simulink model "FCEvReferenceApplication"  (R2022a)
settings: Solver=VariableStepAuto  StartTime=0  StopTime=2474  RelTol=1e-3  EnableMultiTasking=on
undefined symbols (not defined in the file or in its folder): GenerateMappedFuelCellCalibrations
libraries: autolibshared x2
settings Model: DataDictionary=VehicleConfig.sldd  ModifiedByFormat=The MathWorks, Inc.  SimulationMode=accelerator  PauseTimes=0  Creator=The MathWorks, Inc.  LastModifiedBy=The MathWorks, Inc.
settings SolverCC: MaxConsecutiveMinStep=3  ZeroCrossAlgorithm=Adaptive  AlgebraicLoopSolver=TrustRegion  AutoInsertRateTranBlk=on  DecoupledContinuousIntegration=on  MinimalZcImpactIntegration=on  MaxZcPerStep=1
settings DataIOCC: SaveOutput=off  DSMLogging=off  SaveTime=off  ReturnWorkspaceOutputs=off
settings DebuggingCC: UnderspecifiedInitializationDetection=Classic  MergeDetectMultiDrivingBlocksExec=none  IgnoredZcDiagnostic=none  UnconnectedInputMsg=warning  UnconnectedOutputMsg=warning  UnconnectedLineMsg=warning  ModelReferenceExtraNoncontSigs=none  PregeneratedLibrarySubsystemCodeDiagnostic=none  SFMachineParentedDataDiag=warning  ArithmeticOperatorsInVariantConditions=warning
settings ModelReferenceCC: UpdateModelReferenceTargets=IfOutOfDate  ModelReferenceMinAlgLoopOccurrences=on  PropagateSignalLabelsOutOfModel=off
settings SFSimCC: SimUseLocalCustomCode=off
settings RTWCC: RTWUseLocalCustomCode=off  DLArmComputeVersion=19.05
settings CodeAppCC: StateflowObjectComments=on
settings GRTTargetCC: TargetLangStandard=C89/C90 (ANSI)
settings ConfigComp: CovMetricSettings=dsw  CovSaveCumulativeToWorkspaceVar=on  CovSaveSingleToWorkspaceVar=on  CovExternalEMLEnable=off

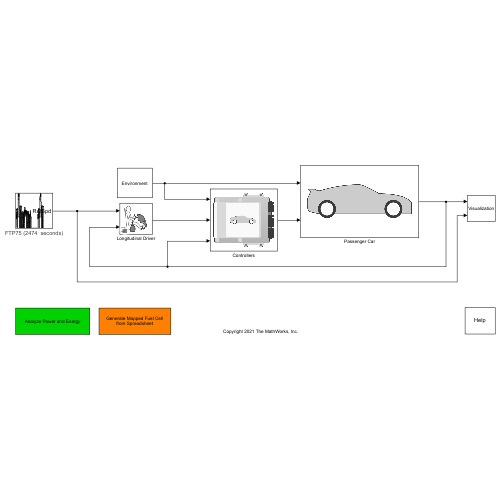
[thumbnail: Simulink's stored preview of the top-level diagram]
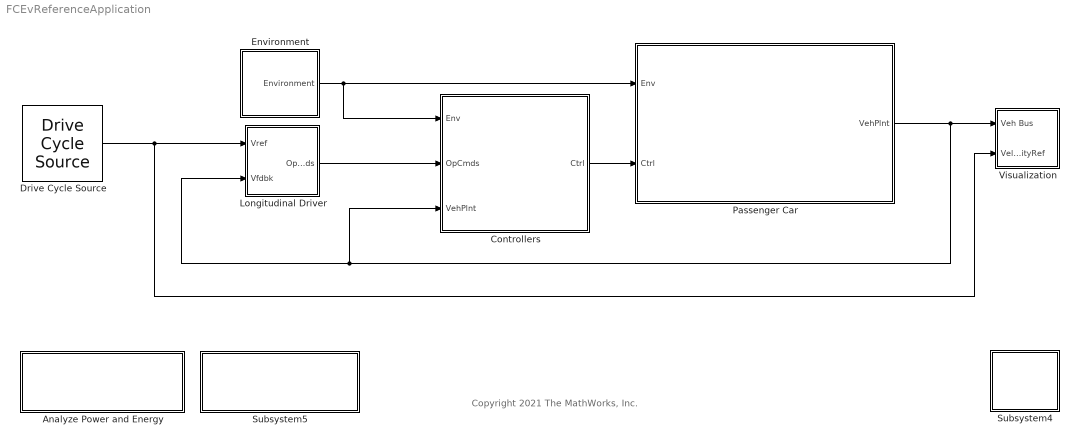
== system FCEvReferenceApplication ==
  note: Copyright 2021 The MathWorks, Inc.
  Analyze Power and Energy : Subsystem
      settings: OpenFcn=edit GenerateEnergyReport
      mask Display: disp(getString(message('autoblks:autoblkVehMask:powAndEne')))
  Controllers : Subsystem
      mask Display: image('SystemControllers.png','center')
  Drive Cycle Source : autolibshared/Drive Cycle Source  cycleVar=FTP75  fileVar=L:\Bauto\matlab\test\toolbox\shared\autoblks\scenario\adac.txt  tfinal="2474  seconds"  cycleRepeat=off  outAccPort=off  outGearPort=off  gearList=No gear data  t_wot1=1  xdot_woto=0  xdot_wot1=26.8  t_wot2=30  xdot_wot2=0  t_wotend=40  srcUnit=m/s  outUnit=m/s  srcAccUnit=m/s/s  outAccUnit=m/s^2  dt=0  aMode=1  faultOption=off  velBnd=2  velBndUnit=mph  inUnit=m/s  timeBnd=1  failOption=off  stopSim=off  maxFaultCnt=10  maxFaultTime=2  maxTotFaultTime=15  traceOption=off  dtTrace=1  traceWindow=10  lastDCname=FTP75  lastOutUnit=mph  lastDT=0  lastTB=1  lastSB=2  forceCalcBound=off
      settings: SourceProductBaseCode=PW,DR,MT,VE
  Environment : Subsystem
      mask Display: disp(getString(message('autoblks:autoblkVehMask:environ')))
  Longitudinal Driver : Subsystem  Variant=on  VariantControlMode=label  VariantControl=Variant1  LabelModeActiveChoice=0
      mask Display:
      | if strcmp('1',get_param(gcb,'ActiveVariant'))
      |     disp('Open Loop')
      | else
      |     image('LongitudinalDriver.png','center');
      | end
  Passenger Car : Subsystem
      mask Display: image('PassengerVehicle.png','center')
  Subsystem4 : Subsystem
      settings: OpenFcn=helpview([docroot,'/toolbox/autoblks/helptargets.map'], 'fcev_refapp')
      mask Display: disp(getString(message('autoblks:autoblkVehMask:help')))
  Subsystem5 : Subsystem  LoadFcn=GenerateMappedFuelCellCalibrations(gcb, 'CheckMBCLicense');  mask(Generate Mapped Fuel Cell from Spreadsheet){SpreadsheetFileName=FuelCellPerformanceData.xlsx, MBCProjectName=MappedFuelCell.mat, CageFileName=MappedFuelCell.cag, MappedFCellMdlRefName=FCElectricPlant}
      mask prompts: SpreadsheetFileName "autoblks:autoblkMappedFuelCellMask:mapSheetFile"; MBCProjectName "autoblks:autoblkMappedFuelCellMask:mbcProj"; CageFileName "autoblks:autoblkMappedFuelCellMask:cageFile"; MappedFCellMdlRefName "autoblks:autoblkMappedFuelCellMask:mappedEng"
      mask help: autoblks:autoblkMappedFuelCellMask:descSheet
      mask init:
      | GenerateMappedFuelCellCalibrations(gcb, 'Init');
      settings: OpenFcn=open_system(gcb, 'mask')
      mask Help: helpview([docroot,'/toolbox/autoblks/helptargets.map'], 'fcev_mapped_spreadsheet')
      mask DialogControl DescTextVar Prompt: autoblks:autoblkMappedFuelCellMask:descSheet
      mask DialogControl MBCHyperlink Prompt: autoblks:autoblkMappedFuelCellMask:reqOpt
      mask DialogControl MBCHyperlink Callback: helpview([docroot,'/toolbox/autoblks/helptargets.map'], 'siengine_dyno_refapp')
      mask DialogControl Container3 Prompt: autoblks:autoblkMappedFuelCellMask:step1
      mask DialogControl SpreadsheetFileName Prompt: Spreadsheet file:
      mask DialogControl SpreadsheetFileNameSelect Prompt: autoblks:autoblkMappedFuelCellMask:ellipsis
      mask DialogControl SpreadsheetFileNameSelect Callback: GenerateMappedFuelCellCalibrations(gcb, 'SpreadsheetFileNameSelect');
      mask DialogControl GenMappedFCellCalButton Prompt: autoblks:autoblkMappedFuelCellMask:fcellCal
      mask DialogControl GenMappedFCellCalButton Callback: GenerateMappedFuelCellCalibrations(gcb, 'GenMappedFCellCalButton');
      mask DialogControl MBCProjectName Prompt: MBC project name:
      mask DialogControl CageFileName Prompt: CAGE file name:
      mask DialogControl Container4 Prompt: autoblks:autoblkMappedFuelCellMask:step2
      mask DialogControl ApplyCalMappedFCellButton Prompt: autoblks:autoblkMappedFuelCellMask:applyCal
      mask DialogControl ApplyCalMappedFCellButton Callback: GenerateMappedFuelCellCalibrations(gcb, 'ApplyCalMappedFCellButton');
      mask Display: disp(getString(message('autoblks:autoblkMappedFuelCellMask:mapSpreadLabel')))
  Visualization : Subsystem
      mask Display: disp(getString(message('autoblks:autoblkVehMask:visual')))
  wires:
  Longitudinal Driver/1(" OpCmds") -> Controllers/2(OpCmds)
  Drive Cycle Source/1 -> Longitudinal Driver/1("Vref "), Visualization/2(VelocityRef)
  Environment/1(Environment) -> Controllers/1(Env), Passenger Car/1(Env)
  Controllers/1(Ctrl) -> Passenger Car/2(Ctrl)
  Passenger Car/1(VehPlnt) -> Controllers/3(VehPlnt), Longitudinal Driver/2("Vfdbk "), Visualization/1(Veh Bus)

== system FCEvReferenceApplication/Analyze Power and Energy ==

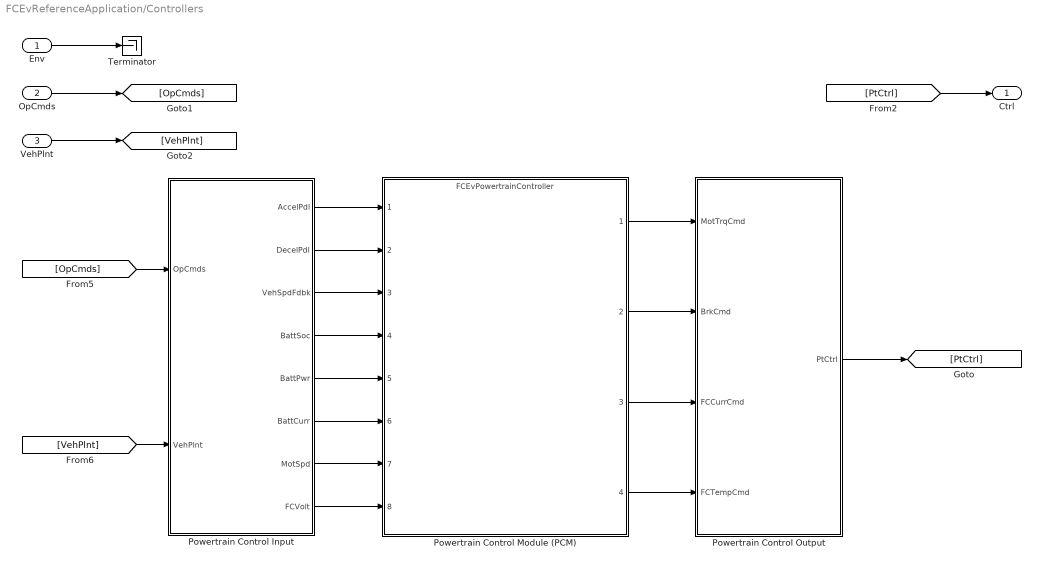
== system FCEvReferenceApplication/Controllers ==
  Env : Inport
  OpCmds : Inport  Port=2
  VehPlnt : Inport  Port=3
  Powertrain Control Input : Subsystem
  Powertrain Control Module (PCM) : ModelReference  ModelNameDialog=FCEvPowertrainController.slx  ModelReferenceVersion=4.1
  Powertrain Control Output : Subsystem
  Terminator : Terminator
  Ctrl : Outport  VectorParamsAs1DForOutWhenUnconnected=off
  wires:
  [OpCmds] -> Powertrain Control Input/1(OpCmds)
  Powertrain Control Input/6(BattCurr) -> Powertrain Control Module (PCM)/6
  Powertrain Control Module (PCM)/4 -> Powertrain Control Output/4(FCTempCmd)
  VehPlnt/1 -> [VehPlnt]
  Powertrain Control Input/2(DecelPdl) -> Powertrain Control Module (PCM)/2
  Powertrain Control Input/3(VehSpdFdbk) -> Powertrain Control Module (PCM)/3
  Powertrain Control Input/5(BattPwr) -> Powertrain Control Module (PCM)/5
  Powertrain Control Input/8(FCVolt) -> Powertrain Control Module (PCM)/8
  [PtCtrl] -> Ctrl/1
  [VehPlnt] -> Powertrain Control Input/2(VehPlnt)
  OpCmds/1 -> [OpCmds]
  Powertrain Control Input/4(BattSoc) -> Powertrain Control Module (PCM)/4
  Powertrain Control Module (PCM)/3 -> Powertrain Control Output/3(FCCurrCmd)
  Powertrain Control Module (PCM)/1 -> Powertrain Control Output/1(MotTrqCmd)
  Powertrain Control Module (PCM)/2 -> Powertrain Control Output/2(BrkCmd)
  Powertrain Control Input/7(MotSpd) -> Powertrain Control Module (PCM)/7
  Env/1 -> Terminator/1
  Powertrain Control Input/1(AccelPdl) -> Powertrain Control Module (PCM)/1
  Powertrain Control Output/1(PtCtrl) -> [PtCtrl]

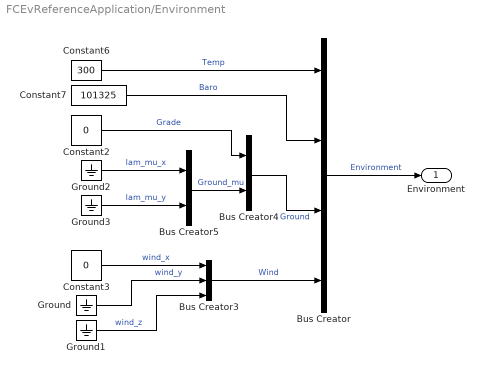
== system FCEvReferenceApplication/Environment ==
  Bus Creator : BusCreator  Inputs=4
  Bus Creator3 : BusCreator  Inputs=3
  Bus Creator4 : BusCreator  Inputs=2
  Bus Creator5 : BusCreator  Inputs=2
  Constant2 : Constant  Value=0
  Constant3 : Constant  Value=0
  Constant6 : Constant  Value=300
  Constant7 : Constant  Value=101325
  Ground{,1..3} (4 alike) : Ground
  Environment : Outport  VectorParamsAs1DForOutWhenUnconnected=off
  wires:
  Ground2/1 -> Bus Creator5/1  "lam_mu_x"
  Ground3/1 -> Bus Creator5/2  "lam_mu_y"
  Bus Creator5/1 -> Bus Creator4/2  "Ground_mu"
  Bus Creator4/1 -> Bus Creator/3  "Ground"
  Bus Creator3/1 -> Bus Creator/4  "Wind"
  Constant3/1 -> Bus Creator3/1  "wind_x"
  Ground/1 -> Bus Creator3/2  "wind_y"
  Ground1/1 -> Bus Creator3/3  "wind_z"
  Constant6/1 -> Bus Creator/1  "Temp"
  Constant2/1 -> Bus Creator4/1  "Grade"
  Bus Creator/1 -> Environment/1  "Environment"
  Constant7/1 -> Bus Creator/2  "Baro"

== system FCEvReferenceApplication/Longitudinal Driver ==
  note: To switch variants, right-click on this subsystem (from one level above) and chose:
      | Variant, Active choice, <your selection>
  "Vref " : Inport
  "Vfdbk " : Inport  Port=2
  Longitudinal Driver : Subsystem  VariantControl=0
      mask Display: image('LongitudinalDriver.png', 'center')
  Open Loop : Subsystem  VariantControl=1
      mask Display: disp('Open Loop')
  " OpCmds" : Outport  VectorParamsAs1DForOutWhenUnconnected=off

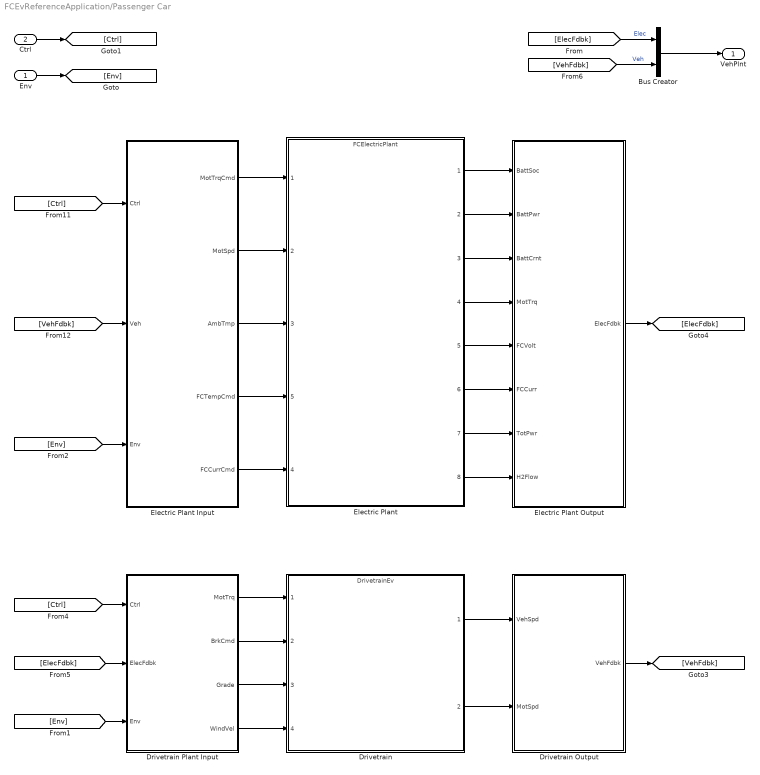
== system FCEvReferenceApplication/Passenger Car ==
  Env : Inport
  Ctrl : Inport  Port=2
  Bus Creator : BusCreator  Inputs=2
  Drivetrain : ModelReference  ModelNameDialog=DrivetrainEv.slx  ModelReferenceVersion=6.1
  Drivetrain Output : Subsystem
  Drivetrain Plant Input : Subsystem
  Electric Plant : ModelReference  ModelNameDialog=FCElectricPlant.slx  ModelReferenceVersion=4.151
      settings: PortSchema="{\"entries\":[{\"content\":{\"sides\":[{\"content\":{\"connectorIds\":[\"In1\",\"In2\",\"In3\",\"In5\",\"In4\"]},\"type\":\"ConnectorPlacement.EquallySpacedRectSide\",\"uuid\":\"252331aa-c2e1-4212-91c7-54a4f8807c1b\"},{\"content\":{\"connectorIds\":[\"Out1\",\"Out2\",\"Out3\",\"Out4\",\"Out5\",\"Out6\",\"Out7\",\"Out8\"],\"side\":\"RIGHT\"},\"type\":\"ConnectorPlacement.EquallySpacedRectSide\",\"uuid\":\"96a2e807-7b6e-43c6-b371-83afbf277557\"},{\"content\":{\"connectorIds\":[],\"side\":\"TOP\"},\"type\":\"ConnectorPlacement.EquallySpacedRectSide\",\"uuid\":\"573edb4a-38fa-4d49-8fd7-93dca65813a5\"}]},\"type\":\"ConnectorPlacement.EquallySpacedConnector\",\"uuid\":\"acfa41e8-7930-436b-acd7-e14a4a7fb9aa\"}],\"packageUris\":[\"http://schema.mathworks.com/mf0/Connector/R2020b\"],\"version\":\"1.0\"}"
  Electric Plant Input : Subsystem
  Electric Plant Output : Subsystem
  VehPlnt : Outport  VectorParamsAs1DForOutWhenUnconnected=off
  wires:
  Electric Plant/1 -> Electric Plant Output/1(BattSoc)
  Env/1 -> [Env]
  Electric Plant/6 -> Electric Plant Output/6(FCCurr)
  Electric Plant/5 -> Electric Plant Output/5(FCVolt)
  Electric Plant/3 -> Electric Plant Output/3(BattCrnt)
  Electric Plant/4 -> Electric Plant Output/4(MotTrq)
  Bus Creator/1 -> VehPlnt/1
  [ElecFdbk] -> Bus Creator/1  "Elec"
  Electric Plant Output/1(ElecFdbk) -> [ElecFdbk]
  [Env] -> Electric Plant Input/3(Env)
  Electric Plant Input/4(FCTempCmd) -> Electric Plant/5
  Electric Plant Input/2(MotSpd) -> Electric Plant/2
  Electric Plant Input/1(MotTrqCmd) -> Electric Plant/1
  Electric Plant/2 -> Electric Plant Output/2(BattPwr)
  [VehFdbk] -> Bus Creator/2  "Veh"
  Electric Plant Input/5(FCCurrCmd) -> Electric Plant/4
  [Ctrl] -> Electric Plant Input/1(Ctrl)
  Ctrl/1 -> [Ctrl]
  [VehFdbk] -> Electric Plant Input/2(Veh)
  Electric Plant Input/3(AmbTmp) -> Electric Plant/3
  Drivetrain/1 -> Drivetrain Output/1(VehSpd)
  Drivetrain Plant Input/2(BrkCmd) -> Drivetrain/2
  Drivetrain Output/1(VehFdbk) -> [VehFdbk]
  [Ctrl] -> Drivetrain Plant Input/1(Ctrl)
  Drivetrain Plant Input/1(MotTrq) -> Drivetrain/1
  [Env] -> Drivetrain Plant Input/3(Env)
  Drivetrain Plant Input/4(WindVel) -> Drivetrain/4
  Drivetrain Plant Input/3(Grade) -> Drivetrain/3
  Drivetrain/2 -> Drivetrain Output/2(MotSpd)
  [ElecFdbk] -> Drivetrain Plant Input/2(ElecFdbk)
  Electric Plant/7 -> Electric Plant Output/7(TotPwr)
  Electric Plant/8 -> Electric Plant Output/8(H2Flow)

== system FCEvReferenceApplication/Subsystem4 ==

== system FCEvReferenceApplication/Subsystem5 ==

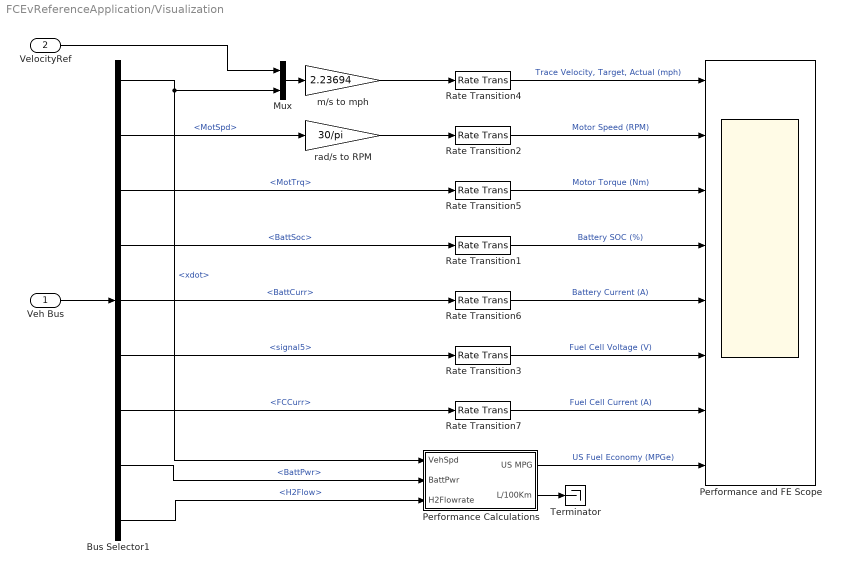
== system FCEvReferenceApplication/Visualization ==
  Veh Bus : Inport
  VelocityRef : Inport  Port=2
  Bus Selector1 : BusSelector  OutputSignals=Veh.xdot,Veh.MotSpd,Elec.MotTrq,Elec.BattSoc,Elec.BattCurr,Elec.signal5,Elec.FCCurr,Elec.BattPwr,Elec.H2Flow
  Mux : Mux  Inputs=2
  Performance Calculations : Subsystem
  Performance and FE Scope : Scope  NumInputPorts=8
  Rate Transition{1..7} (7 alike) : RateTransition  Deterministic=off
  Terminator : Terminator
  m/s to mph : Gain  Gain=2.23694
  rad/s to RPM : Gain  Gain=30/pi
  wires:
  Veh Bus/1 -> Bus Selector1/1
  Bus Selector1/1 -> Performance Calculations/1(VehSpd), Mux/2  "<xdot>"
  Mux/1 -> m/s to mph/1
  Performance Calculations/1(US MPG) -> Performance and FE Scope/8  "US Fuel Economy (MPGe)"
  Performance Calculations/2(L/100Km) -> Terminator/1
  m/s to mph/1 -> Rate Transition4/1
  Bus Selector1/4 -> Rate Transition1/1  "<BattSoc>"
  VelocityRef/1 -> Mux/1
  Rate Transition1/1 -> Performance and FE Scope/4  "Battery SOC (%)"
  Rate Transition2/1 -> Performance and FE Scope/2  "Motor Speed (RPM)"
  Rate Transition4/1 -> Performance and FE Scope/1  "Trace Velocity, Target, Actual (mph)"
  Bus Selector1/2 -> rad/s to RPM/1  "<MotSpd>"
  Bus Selector1/8 -> Performance Calculations/2(BattPwr)  "<BattPwr>"
  rad/s to RPM/1 -> Rate Transition2/1
  Bus Selector1/3 -> Rate Transition5/1  "<MotTrq>"
  Rate Transition5/1 -> Performance and FE Scope/3  "Motor Torque (Nm)"
  Rate Transition6/1 -> Performance and FE Scope/5  "Battery Current (A)"
  Bus Selector1/5 -> Rate Transition6/1  "<BattCurr>"
  Bus Selector1/9 -> Performance Calculations/3(H2Flowrate)  "<H2Flow>"
  Bus Selector1/7 -> Rate Transition7/1  "<FCCurr>"
  Rate Transition7/1 -> Performance and FE Scope/7  "Fuel Cell Current (A)"
  Bus Selector1/6 -> Rate Transition3/1  "<signal5>"
  Rate Transition3/1 -> Performance and FE Scope/6  "Fuel Cell Voltage (V)"

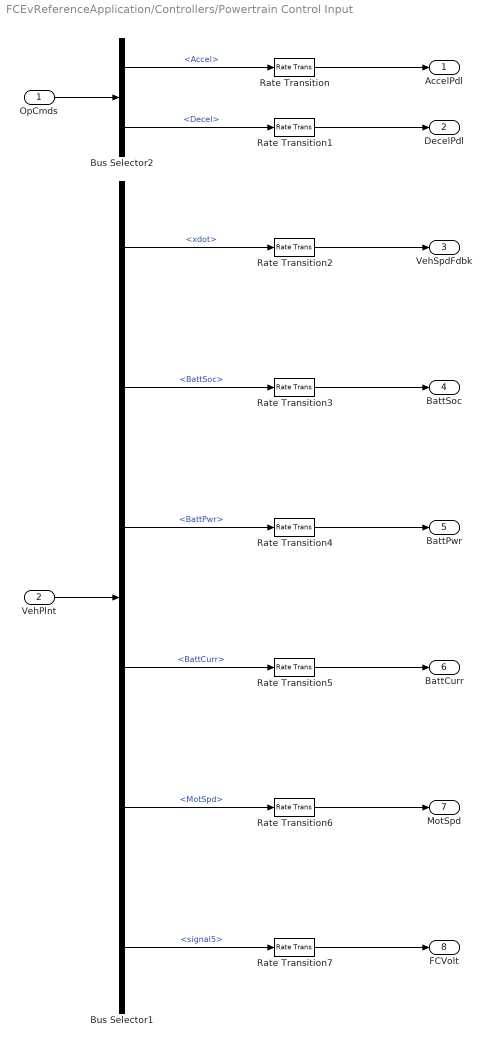
== system FCEvReferenceApplication/Controllers/Powertrain Control Input ==
  OpCmds : Inport
  VehPlnt : Inport  Port=2
  Bus Selector1 : BusSelector  OutputSignals=Veh.xdot,Elec.BattSoc,Elec.BattPwr,Elec.BattCurr,Veh.MotSpd,Elec.signal5
  Bus Selector2 : BusSelector  OutputSignals=Accel,Decel
  Rate Transition{,1..7} (8 alike) : RateTransition  Deterministic=off
  AccelPdl : Outport  VectorParamsAs1DForOutWhenUnconnected=off
  DecelPdl : Outport  Port=2  VectorParamsAs1DForOutWhenUnconnected=off
  VehSpdFdbk : Outport  Port=3  VectorParamsAs1DForOutWhenUnconnected=off
  BattSoc : Outport  Port=4  VectorParamsAs1DForOutWhenUnconnected=off
  BattPwr : Outport  Port=5  VectorParamsAs1DForOutWhenUnconnected=off
  BattCurr : Outport  Port=6  VectorParamsAs1DForOutWhenUnconnected=off
  MotSpd : Outport  Port=7  VectorParamsAs1DForOutWhenUnconnected=off
  FCVolt : Outport  Port=8  VectorParamsAs1DForOutWhenUnconnected=off
  wires:
  OpCmds/1 -> Bus Selector2/1
  VehPlnt/1 -> Bus Selector1/1
  Bus Selector2/1 -> Rate Transition/1  "<Accel>"
  Bus Selector2/2 -> Rate Transition1/1  "<Decel>"
  Bus Selector1/1 -> Rate Transition2/1  "<xdot>"
  Bus Selector1/2 -> Rate Transition3/1  "<BattSoc>"
  Bus Selector1/3 -> Rate Transition4/1  "<BattPwr>"
  Bus Selector1/4 -> Rate Transition5/1  "<BattCurr>"
  Bus Selector1/5 -> Rate Transition6/1  "<MotSpd>"
  Rate Transition/1 -> AccelPdl/1
  Rate Transition1/1 -> DecelPdl/1
  Rate Transition2/1 -> VehSpdFdbk/1
  Rate Transition3/1 -> BattSoc/1
  Rate Transition4/1 -> BattPwr/1
  Rate Transition5/1 -> BattCurr/1
  Rate Transition6/1 -> MotSpd/1
  Rate Transition7/1 -> FCVolt/1
  Bus Selector1/6 -> Rate Transition7/1  "<signal5>"

== system FCEvReferenceApplication/Controllers/Powertrain Control Output ==
  MotTrqCmd : Inport
  BrkCmd : Inport  Port=2
  FCCurrCmd : Inport  Port=3
  FCTempCmd : Inport  Port=4
  Bus Creator : BusCreator  Inputs=4
  PtCtrl : Outport  VectorParamsAs1DForOutWhenUnconnected=off
  wires:
  BrkCmd/1 -> Bus Creator/2  "BrkCmd"
  Bus Creator/1 -> PtCtrl/1  "PtCtrl"
  MotTrqCmd/1 -> Bus Creator/1  "MotTrqCmd"
  FCCurrCmd/1 -> Bus Creator/3  "FCCurrCmd"
  FCTempCmd/1 -> Bus Creator/4  "FCTempCmd"

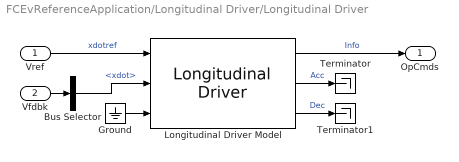
== system FCEvReferenceApplication/Longitudinal Driver/Longitudinal Driver ==
  Vref : Inport
  Vfdbk : Inport  Port=2
  Bus Selector : BusSelector  OutputSignals=Veh.xdot
  Ground : Ground
  Longitudinal Driver Model : autolibshared/Longitudinal Driver  extAccelOvr=off  extDecelOvr=off  extAccelHld=off  extDecelHld=off  extAccelZero=off  extDecelZero=off  cntrlType=Predictive  shftType=Reverse, Neutral, Drive  velUnits=m/s  gearOut=off  Kp=1  Ki=1  Kff=0  Kg=0  VehVelVec=[0 100]  KffVec=[.1 .1]  KpVec=[10 10]  KiVec=[5 5]  KgVec=[0 0]  m=1500  Kpt=10000  tau=0.12  L=4  aR=160  bR=1  cR=0.36  g=9.81  vnom=1  Kaw=0  tauerr=0  tauPt=2  GearInit=0  tShift=.1  pdlVec=[0.1 0.4 0.5 0.9]  upShftTbl=[-1 12.9375 26.4375 39.9375 51.18749999999999 62.4375 72.84375 83.25;-1 16.3125 29.8125 43.3125 54.5624 65.8125 76.78125 87.75;-1 19.6875 33.1875 46.68749999999999 57.9375 69.1875 80.71875 92.25;-1 33 52.5 77.25 100.5 138.75 161.875 185]  dwnShftTbl=[1 9.5625 23.0625 36.5625 47.8125 59.0625 68.90625 78.75;1 12.9375 26.4375 39.9375 51.18749999999999 62.4375 72.84375 83.25;1 16.3125 29.8125 43.3125 54.562499 65.8125 76.78125 87.75;1 19.6875 33.1875 46.68749999999999 57.9375 69.1875 80.71875 92.25]  tClutch=.5  tRev=.5  tPark=120  aMode=1  UpGearVec="[0  1  2  3  4  5  6  7]"  DownGearVec="[1  2  3  4  5  6  7  8]"
      settings: SourceProductBaseCode=PW,DR,MT,VE
  Terminator : Terminator
  Terminator1 : Terminator
  OpCmds : Outport  VectorParamsAs1DForOutWhenUnconnected=off
  wires:
  Bus Selector/1 -> Longitudinal Driver Model/2  "<xdot>"
  Vref/1 -> Longitudinal Driver Model/1  "xdotref"
  Vfdbk/1 -> Bus Selector/1
  Longitudinal Driver Model/2 -> Terminator/1  "Acc"
  Longitudinal Driver Model/3 -> Terminator1/1  "Dec"
  Ground/1 -> Longitudinal Driver Model/3
  Longitudinal Driver Model/1 -> OpCmds/1  "Info"

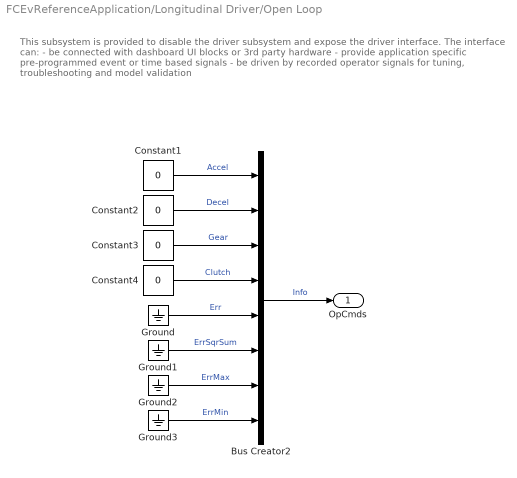
== system FCEvReferenceApplication/Longitudinal Driver/Open Loop ==
  note: This subsystem is provided to disable the driver subsystem and expose the driver interface.
      |
      | The interface can:
      | - be connected with dashboard UI blocks or 3rd party hardware
      | - provide application specific pre-programmed event or time based signals
      | - be driven by recorded operator signals for tuning, troubleshooting and model validation
  Bus Creator2 : BusCreator  Inputs=8
  Constant{1..4} (4 alike) : Constant  Value=0
  Ground{,1..3} (4 alike) : Ground
  OpCmds : Outport  VectorParamsAs1DForOutWhenUnconnected=off
  wires:
  Ground3/1 -> Bus Creator2/8  "ErrMin"
  Ground1/1 -> Bus Creator2/6  "ErrSqrSum"
  Bus Creator2/1 -> OpCmds/1  "Info"
  Ground2/1 -> Bus Creator2/7  "ErrMax"
  Constant1/1 -> Bus Creator2/1  "Accel"
  Constant3/1 -> Bus Creator2/3  "Gear"
  Constant2/1 -> Bus Creator2/2  "Decel"
  Ground/1 -> Bus Creator2/5  "Err"
  Constant4/1 -> Bus Creator2/4  "Clutch"

== system FCEvReferenceApplication/Passenger Car/Drivetrain Output ==
  VehSpd : Inport
  MotSpd : Inport  Port=2
  Bus Creator1 : BusCreator  Inputs=2
  VehFdbk : Outport  VectorParamsAs1DForOutWhenUnconnected=off
  wires:
  Bus Creator1/1 -> VehFdbk/1  "VehFdbk"
  VehSpd/1 -> Bus Creator1/1
  MotSpd/1 -> Bus Creator1/2  "MotSpd"

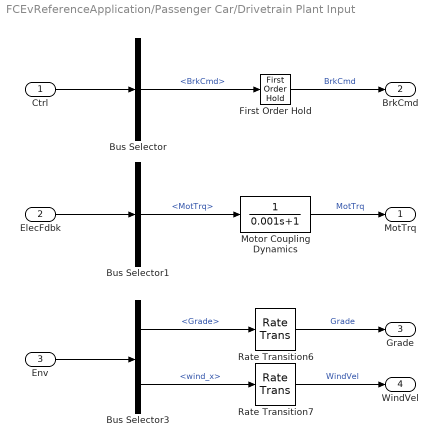
== system FCEvReferenceApplication/Passenger Car/Drivetrain Plant Input ==
  Ctrl : Inport
  ElecFdbk : Inport  Port=2
  Env : Inport  Port=3
  Bus Selector : BusSelector  OutputSignals=BrkCmd
  Bus Selector1 : BusSelector  OutputSignals=MotTrq
  Bus Selector3 : BusSelector  OutputSignals=Ground.Grade,Wind.wind_x
  First Order Hold : FirstOrderHold  ErrorTolerance=inf
  Motor Coupling Dynamics : TransferFcn  Denominator=[0.001 1]
  Rate Transition6 : RateTransition  Deterministic=off
  Rate Transition7 : RateTransition  Deterministic=off
  MotTrq : Outport  VectorParamsAs1DForOutWhenUnconnected=off
  BrkCmd : Outport  Port=2  VectorParamsAs1DForOutWhenUnconnected=off
  Grade : Outport  Port=3  VectorParamsAs1DForOutWhenUnconnected=off
  WindVel : Outport  Port=4  VectorParamsAs1DForOutWhenUnconnected=off
  wires:
  Ctrl/1 -> Bus Selector/1
  Bus Selector/1 -> First Order Hold/1  "<BrkCmd>"
  First Order Hold/1 -> BrkCmd/1  "BrkCmd"
  ElecFdbk/1 -> Bus Selector1/1
  Bus Selector1/1 -> Motor Coupling Dynamics/1  "<MotTrq>"
  Env/1 -> Bus Selector3/1
  Rate Transition6/1 -> Grade/1  "Grade"
  Rate Transition7/1 -> WindVel/1  "WindVel"
  Bus Selector3/1 -> Rate Transition6/1  "<Grade>"
  Bus Selector3/2 -> Rate Transition7/1  "<wind_x>"
  Motor Coupling Dynamics/1 -> MotTrq/1  "MotTrq"

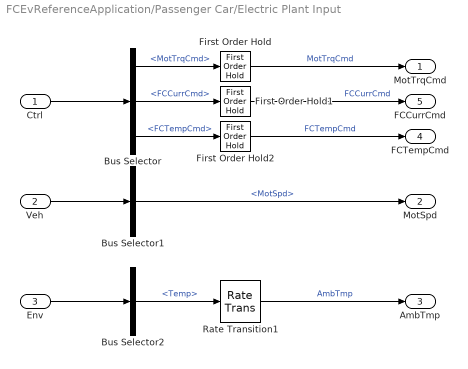
== system FCEvReferenceApplication/Passenger Car/Electric Plant Input ==
  Ctrl : Inport
  Veh : Inport  Port=2
  Env : Inport  Port=3
  Bus Selector : BusSelector  OutputSignals=MotTrqCmd,FCCurrCmd,FCTempCmd
  Bus Selector1 : BusSelector  OutputSignals=MotSpd
  Bus Selector2 : BusSelector  OutputSignals=Temp
  First Order Hold : FirstOrderHold  ErrorTolerance=inf
  First Order Hold1 : FirstOrderHold  ErrorTolerance=inf
  First Order Hold2 : FirstOrderHold  ErrorTolerance=inf
  Rate Transition1 : RateTransition  Deterministic=off
  MotTrqCmd : Outport  VectorParamsAs1DForOutWhenUnconnected=off
  MotSpd : Outport  Port=2  VectorParamsAs1DForOutWhenUnconnected=off
  AmbTmp : Outport  Port=3  VectorParamsAs1DForOutWhenUnconnected=off
  FCTempCmd : Outport  Port=4  VectorParamsAs1DForOutWhenUnconnected=off
  FCCurrCmd : Outport  Port=5  VectorParamsAs1DForOutWhenUnconnected=off
  wires:
  First Order Hold/1 -> MotTrqCmd/1  "MotTrqCmd"
  Ctrl/1 -> Bus Selector/1
  Bus Selector/1 -> First Order Hold/1  "<MotTrqCmd>"
  Veh/1 -> Bus Selector1/1
  Bus Selector1/1 -> MotSpd/1  "<MotSpd>"
  Env/1 -> Bus Selector2/1
  Rate Transition1/1 -> AmbTmp/1  "AmbTmp"
  Bus Selector2/1 -> Rate Transition1/1  "<Temp>"
  Bus Selector/2 -> First Order Hold1/1  "<FCCurrCmd>"
  Bus Selector/3 -> First Order Hold2/1  "<FCTempCmd>"
  First Order Hold1/1 -> FCCurrCmd/1  "FCCurrCmd"
  First Order Hold2/1 -> FCTempCmd/1  "FCTempCmd"

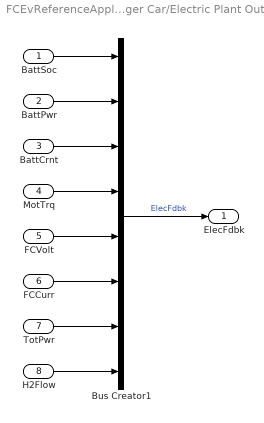
== system FCEvReferenceApplication/Passenger Car/Electric Plant Output ==
  BattSoc : Inport
  BattPwr : Inport  Port=2
  BattCrnt : Inport  Port=3
  MotTrq : Inport  Port=4
  FCVolt : Inport  Port=5
  FCCurr : Inport  Port=6
  TotPwr : Inport  Port=7
  H2Flow : Inport  Port=8
  Bus Creator1 : BusCreator  Inputs=8
  ElecFdbk : Outport  VectorParamsAs1DForOutWhenUnconnected=off
  wires:
  Bus Creator1/1 -> ElecFdbk/1  "ElecFdbk"
  BattPwr/1 -> Bus Creator1/2
  BattSoc/1 -> Bus Creator1/1
  BattCrnt/1 -> Bus Creator1/3
  MotTrq/1 -> Bus Creator1/4
  FCVolt/1 -> Bus Creator1/5
  FCCurr/1 -> Bus Creator1/6
  TotPwr/1 -> Bus Creator1/7
  H2Flow/1 -> Bus Creator1/8

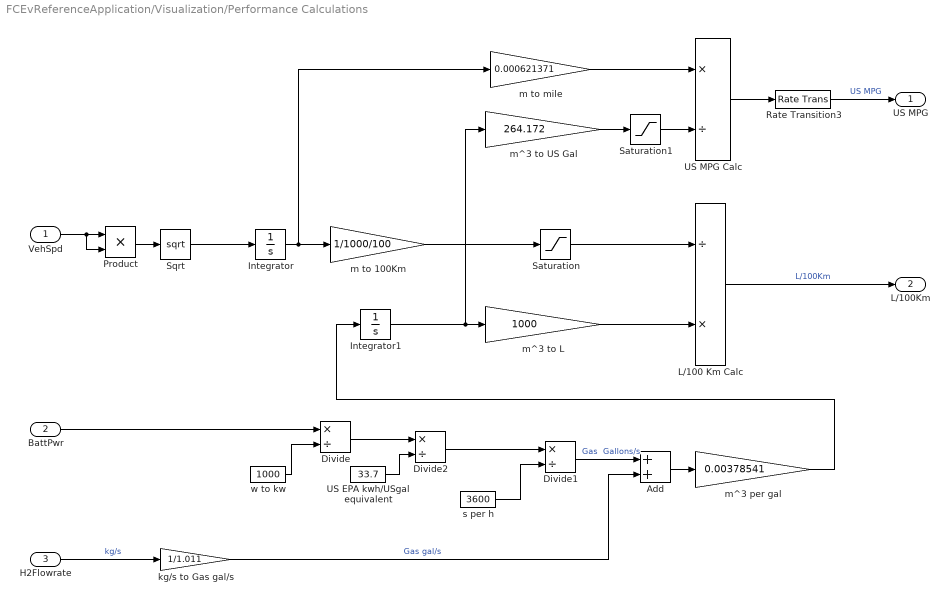
== system FCEvReferenceApplication/Visualization/Performance Calculations ==
  VehSpd : Inport
  BattPwr : Inport  Port=2
  H2Flowrate : Inport  Port=3
  Add : Sum
  Divide : Product  Inputs=*/
  Divide1 : Product  Inputs=*/
  Divide2 : Product  Inputs=*/
  Integrator : Integrator
  Integrator1 : Integrator
  L/100 Km Calc : Product  Inputs=/*
  Product : Product
  Rate Transition3 : RateTransition  Deterministic=off
  Saturation : Saturate  UpperLimit=Inf  LowerLimit=0.001
  Saturation1 : Saturate  UpperLimit=Inf  LowerLimit=1e-3
  Sqrt : Sqrt
  US EPA kwh/USgal equivalent : Constant  Value=33.7
  US MPG Calc : Product  Inputs=*/
  kg/s to Gas gal/s : Gain  Gain=1/1.011
  m to 100Km : Gain  Gain=1/1000/100
  m to mile : Gain  Gain=0.000621371
  m^3 per gal : Gain  Gain=0.00378541
  m^3 to L : Gain  Gain=1000
  m^3 to US Gal : Gain  Gain=264.172
  s per h : Constant  Value=3600
  w to kw : Constant  Value=1000
  US MPG : Outport  VectorParamsAs1DForOutWhenUnconnected=off
  L/100Km : Outport  Port=2  VectorParamsAs1DForOutWhenUnconnected=off
  wires:
  m^3 to US Gal/1 -> Saturation1/1
  m^3 to L/1 -> L/100 Km Calc/2
  Integrator/1 -> m to mile/1, m to 100Km/1
  m to mile/1 -> US MPG Calc/1
  Integrator1/1 -> m^3 to US Gal/1, m^3 to L/1
  Saturation/1 -> L/100 Km Calc/1
  m to 100Km/1 -> Saturation/1
  L/100 Km Calc/1 -> L/100Km/1  "L/100Km"
  US MPG Calc/1 -> Rate Transition3/1
  Saturation1/1 -> US MPG Calc/2
  Rate Transition3/1 -> US MPG/1  "US MPG"
  w to kw/1 -> Divide/2
  Divide/1 -> Divide2/1
  Divide2/1 -> Divide1/1
  s per h/1 -> Divide1/2
  Divide1/1 -> Add/1  "Gas  Gallons/s"
  US EPA kwh/USgal equivalent/1 -> Divide2/2
  BattPwr/1 -> Divide/1
  Sqrt/1 -> Integrator/1
  Product/1 -> Sqrt/1
  VehSpd/1 -> Product/2, Product/1
  m^3 per gal/1 -> Integrator1/1
  H2Flowrate/1 -> kg/s to Gas gal/s/1  "kg/s"
  kg/s to Gas gal/s/1 -> Add/2  "Gas gal/s"
  Add/1 -> m^3 per gal/1
